simulink library "eml_evalin_matlab_lib"  (Simulink 6.0)
settings: Solver=ode45  SolverMode=SingleTasking  StartTime=0.0  StopTime=10.0  RelTol=1e-3
values from neighbouring files (symbols this model uses):
  i = varargin{1}    [sf_mandel_gui.m]
undefined symbols (not defined in the file or in its folder): eml_do_selective_run, sf
settings Model: CovMetricSettings=dcmtr  Creator=The MathWorks Inc.  LastModifiedBy=batserve  ExtModeAutoUpdateStatusClock=off  ProdHWDeviceType=Specified
settings DataIOCC: SignalLoggingName=logsOut
settings OptimizationCC: BooleanDataType=off
settings DebuggingCC: CheckExecutionContextPreStartOutputMsg=on  CheckExecutionContextRuntimeOutputMsg=on  SolverPrmCheckMsg=none
settings HardwareCC: ProdHWDeviceType=Specified  TargetUnknown=on
settings ModelReferenceCC: UpdateModelReferenceTargets=IfOutOfDate

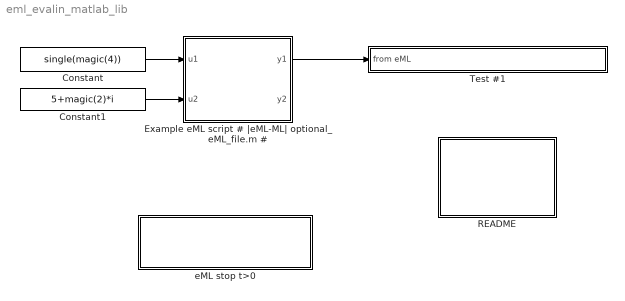
== system eml_evalin_matlab_lib ==
  Constant : Constant  Value=single(magic(4))
  Constant1 : Constant  Value=5+magic(2)*i
  Example eML script # |eML-ML| optional_eML_file.m # : Stateflow chart  PropExecContextAcrossSSBoundary=on
  README : Subsystem  PropExecContextAcrossSSBoundary=on  mask(DocBlock){ECoderFlag=, DocumentType=Text}
      mask prompts: ECoderFlag "E Coder Flag"; DocumentType "Document Type"
      mask help: Use this block to save long descriptive text with the model. Double-clicking the block will open an editor.
      settings: CopyFcn=docblock('breaklink',gcb);  DeleteFcn=docblock('close_document',gcb);  PreSaveFcn=docblock('save_document',gcb);  OpenFcn=docblock('edit_document',gcb);
      mask StyleString: edit,popup(Text|RTF|HTML)
      mask Display:
      | plot([.8 0 0 1 1 .8 .8 1],[1 1 0 0 .8 1 .8 .8]);
      | text(.5,.5,'DOC','horizontalalignment','center');
  Test #1 : Subsystem  InitFcn=|  StopFcn=set_param(gcb,'BackgroundColor','cyan');  PropExecContextAcrossSSBoundary=on  mask(|eML-ML| <= Tol){expected=, emlSource="eml_evalin_matlab_lib/passthrough.y1 in eML Script"(#27), emlBlock=|, tol=0, precision=0, tolPCWIN=[1,1], tolGLNX86=[1,1], tolSOL2=[1,1], tolMAC=[1,1], geck=0}
      | set_param(gcb,'BackgroundColor','orange');             
      |                                                        
      |                                                        
      | if(exist('DO_EML_SINGLE', 'var') && DO_EML_SINGLE == 1)
      |     set_param(gcb, 'precision', '2');                  
      | else                                                   
      |     set_param(gcb, 'precision', '1');                  
      | end
      mask emlBlock=|
      | eml_evalin_matlab_lib/Example
      | eML script
      | ## eML EVALIN MATLAB ##
      mask prompts: tolPCWIN "Tolerance [double single] (Inf disables assertion)"; tolGLNX86 "GLNX86 Tolerance override"; tolSOL2 "SOL2 Tolerance override"; tolMAC "MAC Tolerance override"; geck "Geck (non-zero value disables assertion)"
      mask init:
      | tol = sf('Private','eml_evalin_matlab','tol_calc',tolPCWIN,tolGLNX86,tolSOL2,tolMAC);
      mask Display: disp(sf('Private','eml_evalin_matlab','icon',tol,geck))
  eML stop t>0 : Subsystem  Tag=eML_evalin_testController  InitFcn=set_param(gcb,'BackgroundColor','orange');  StartFcn=eml_do_selective_run('close');  StopFcn=set_param(gcb,'BackgroundColor','cyan');  PropExecContextAcrossSSBoundary=on  mask(eML STOP at T==?){evalinMode=Verbose, stopTime=0, rebuildAll=on}
      mask prompts: evalinMode "eML Evalin Mode"; stopTime "Stop Time (s)"; rebuildAll "Rebuild Everytime"
      mask help: %disp(sf('Private','eml_evalin_matlab','eMLstop'));
      settings: OpenFcn=eml_do_selective_run;
      mask StyleString: popup(Verbose|InBaT|Silent),edit,checkbox
      mask Display: disp('Double-click here first');
  wires:
  Constant/1 -> Example eML script # |eML-ML| optional_eML_file.m #/1(u1)
  Constant1/1 -> Example eML script # |eML-ML| optional_eML_file.m #/2(u2)
  Example eML script # |eML-ML| optional_eML_file.m #/1(y1) -> Test #1/1(from eML)

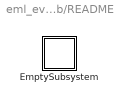
== system eml_evalin_matlab_lib/README ==
  EmptySubsystem : Subsystem  PropExecContextAcrossSSBoundary=on

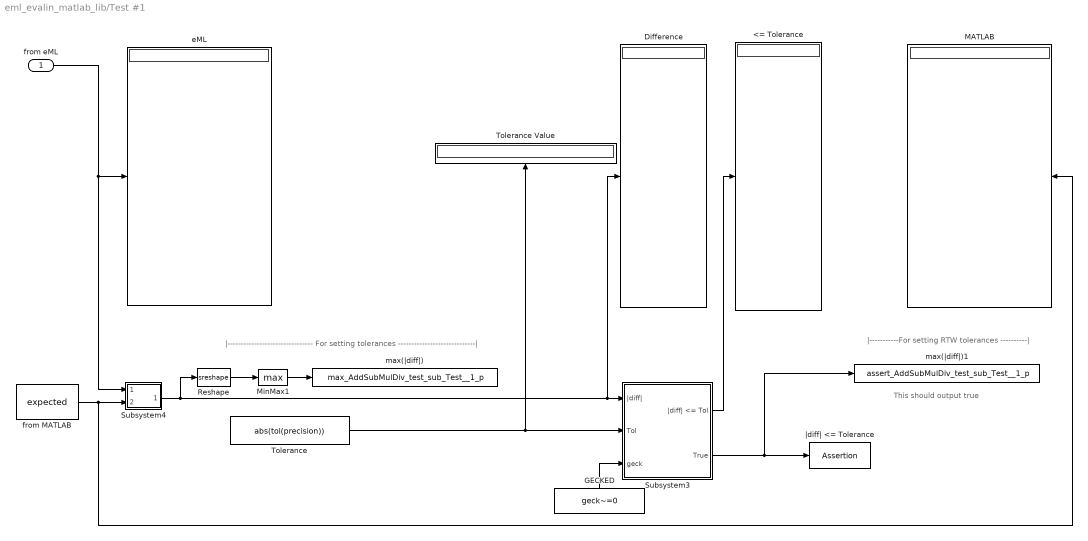
== system eml_evalin_matlab_lib/Test #1 ==
  note: |-----------For setting RTW tolerances ----------|
  note: |-------------------------------- For setting tolerances -----------------------------|
  note: This should output true
  from eML : Inport  Port=1  LatchInput=off
  <= Tolerance : Display
  Difference : Display
  GECKED : Constant  Orientation=up  Value=geck~=0
  MATLAB : Display
  MinMax1 : MinMax  Function=max  SaturateOnIntegerOverflow=on  InputSameDT=on
  Reshape : S-Function  DialogController=Simulink.DDGSource  FunctionName=sreshape  Parameters=OutputDimensionality, OutputDimensions  mask(Reshape){OutputDimensionality=1-D array, OutputDimensions=[1,1]}
      mask prompts: OutputDimensionality "Output dimensionality:"; OutputDimensions "Output dimensions:"
      mask help:
      | Change the dimensions of a vector or matrix input signal. Output
      |  - a one-dimensional array (vector),
      |  - a column vector (Mx1 matrix),
      |  - a row vector (1xN matrix), or
      |  - a matrix or vector with specified dimensions, e.g., [M, N] or [W].
      mask init:
      | s = reshapemask(gcb,'init');
      mask StyleString: popup(1-D array|Column vector|Row vector|Customize),edit
      mask CallbackString: reshapemask(gcb,'cbDimensionality')|
      mask Display: disp('U( : )')
  Subsystem3 : Subsystem  PropExecContextAcrossSSBoundary=on
  Subsystem4 : Subsystem  PropExecContextAcrossSSBoundary=on
      mask Display: disp('|diff|')
  Tolerance : Constant  Value=abs(tol(precision))
  Tolerance Value : Display
      settings: Orientation=up
  eML : Display
  from MATLAB : Constant  Value=expected  VectorParams1D=off
  max(|diff|) : ToWorkspace  VariableName=max_AddSubMulDiv_test_sub_Test__1_p  SampleTime=-1  SaveFormat=Structure
      settings: InitFcn=|
      | if(exist('SET_TOL', 'var') & SET_TOL==1)
      | evalin('base',  ['if(~exist(''max_' strrep(strrep(strrep(gcs, '/', '_'), ' ', '_'), '#', '_') '_p1'')), ' 'max_' strrep(strrep(strrep(gcs, '/', '_'), ' ', '_'), '#', '_') '_p1.signals.values = inf; end'])
      | 
      | evalin('base',  ['if(~exist(''max_' strrep(strrep(strrep(gcs, '/', '_'), ' ', '_'), '#', '_') '_p2'')), max_' strrep(strrep(strrep(gcs, '/', '_'), ' ', '_'), '#', '_') '_p2.signals.values = inf; end'])
      | end
      | 
      | if(exist('EML_NO_OUT', 'var') & EML_NO_OUT==1)
      | set_param(gcb, 'variableName', ['foo_' strrep(strrep(strrep(gcs, '/', '_'), ' ', '_'), '#', '_') '_p' get_param(gcs, 'precision')]);
      | else
      | set_param(gcb, 'variableName', ['max_' strrep(strrep(strrep(gcs, '/', '_'), ' ', '_'), '#', '_') '_p' get_param(gcs, 'precision')]);
      | end
      settings: StopFcn=|
      | if(exist('SET_TOL', 'var') & SET_TOL==1)
      | 
      | 
      | 
      | 
      | 
      | set_param(gcs, ['tol' upper(computer)], ['[' num2str(eval(['max_' strrep(strrep(strrep(gcs, '/', '_'), ' ', '_'), '#', '_') '_p1.signals.values']), '%0.6g') ',' num2str(eval(['max_' strrep(strrep(strrep(gcs, '/', '_'), ' ', '_'), '#', '_') '_p2.signals.values']), '%0.6g') ']'])
      | 
      | 
      | end
      | 
      |                                                                                                                                                                     if(exist('EML_NO_OUT', 'var') & EML_NO_OUT==1)
      | 
      | 
      | 
      | incEmlTol(['max_' strrep(strrep(strrep(gcs, '/', '_'), ' ', '_'), '#', '_') '_p1'])
      | 
      | 
      | incEmlTol(['max_' strrep(strrep(strrep(gcs, '/', '_'), ' ', '_'), '#', '_') '_p2'])
      | 
      | 
      | 
      | end
  max(|diff|)1 : ToWorkspace  VariableName=assert_AddSubMulDiv_test_sub_Test__1_p  SampleTime=-1  SaveFormat=Structure
      settings: InitFcn=set_param(gcb, 'variableName', ['assert_' strrep(strrep(strrep(gcs, '/', '_'), ' ', '_'), '#', '_') '_p' get_param(gcs, 'precision')]);
      settings: StopFcn=|
      | if(exist('SET_TOL', 'var') & SET_TOL==1)
      | set_param(gcs, ['tol' upper(computer)], ['[' num2str(eval(['max_' strrep(strrep(strrep(gcs, '/', '_'), ' ', '_'), '#', '_') '_p1.signals.values']), '%.17g') ',' num2str(eval(['max_' strrep(strrep(strrep(gcs, '/', '_'), ' ', '_'), '#', '_') '_p2.signals.values']), '%.17g') ']'])
      | end
  |diff| <= Tolerance : Assertion  Enabled=off  AssertionFailFcn=sf('Private','eml_evalin_matlab','failure')
  wires:
  GECKED/1 -> Subsystem3/3(geck)
  Subsystem4/1(Abs Diff) -> Difference/1, Subsystem3/1(|diff|), Reshape/1
  Subsystem3/1(|diff| <= Tol) -> <= Tolerance/1
  from MATLAB/1 -> MATLAB/1, Subsystem4/2(In2)
  Subsystem3/2(True) -> |diff| <= Tolerance/1, max(|diff|)1/1
  MinMax1/1 -> max(|diff|)/1
  from eML/1 -> eML/1, Subsystem4/1(In1)
  Reshape/1 -> MinMax1/1
  Tolerance/1 -> Subsystem3/2(Tol), Tolerance Value/1

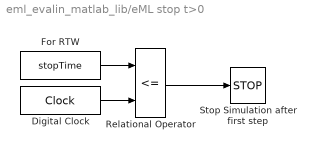
== system eml_evalin_matlab_lib/eML stop t>0 ==
  Digital Clock : DigitalClock
  For RTW : Constant  Value=stopTime
  Relational Operator : RelationalOperator  Operator=<=
  Stop Simulation after first step : Stop
  wires:
  Digital Clock/1 -> Relational Operator/2
  For RTW/1 -> Relational Operator/1
  Relational Operator/1 -> Stop Simulation after first step/1

== system eml_evalin_matlab_lib/README/EmptySubsystem ==

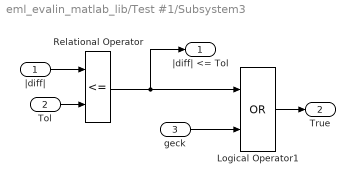
== system eml_evalin_matlab_lib/Test #1/Subsystem3 ==
  |diff| : Inport  Port=1  LatchInput=off
  Tol : Inport  Port=2  LatchInput=off
  geck : Inport  Port=3  LatchInput=off
  Logical Operator1 : Logic  Operator=OR  AllPortsSameDT=off
  Relational Operator : RelationalOperator  Operator=<=  ZeroCross=off
  |diff| <= Tol : Outport
  True : Outport  Port=2
  wires:
  geck/1 -> Logical Operator1/2
  Relational Operator/1 -> Logical Operator1/1, |diff| <= Tol/1
  |diff|/1 -> Relational Operator/1
  Tol/1 -> Relational Operator/2
  Logical Operator1/1 -> True/1

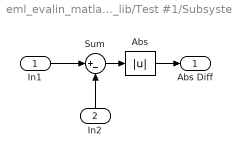
== system eml_evalin_matlab_lib/Test #1/Subsystem4 ==
  In1 : Inport  Port=1  LatchInput=off
  In2 : Inport  Orientation=up  Port=2  LatchInput=off
  Abs : Abs  SaturateOnIntegerOverflow=on
  Sum : Sum  Inputs=|+-  SaturateOnIntegerOverflow=on
  Abs Diff : Outport
  wires:
  Sum/1 -> Abs/1
  In1/1 -> Sum/1
  In2/1 -> Sum/2
  Abs/1 -> Abs Diff/1

== matlab function Example eML script # |eML-ML| optional_eML_file.m # ==
  data: u1 input single size=[4,4]; y1 output single size=[4,4]; u2 input double size=[2,2]; y2 output double size=[2,2]
function [y1,y2]=passthrough(u1,u2)
% a simple pass through example
   y1 = u1;
   y2 = u2;
